simulink model "ModelanfisD"  (R2017a)
settings: Solver=VariableStepAuto  StartTime=0.0  StopTime=578  RelTol=1e-3
values from neighbouring files (symbols this model uses):
  dinneg12 = [-0.01 -0.01 -0.02 -0.01 -0.01 -0.01 0 0 0 0 0.01 -0.01 ... (2312 elements, 578x4)]    [anfisd.mat]    (also in anfisfin.mat; cinco.mat)
libraries: dspsrcs4 x77, fuzblock x22
settings Model: Creator=Dell  LastModifiedBy=Dell

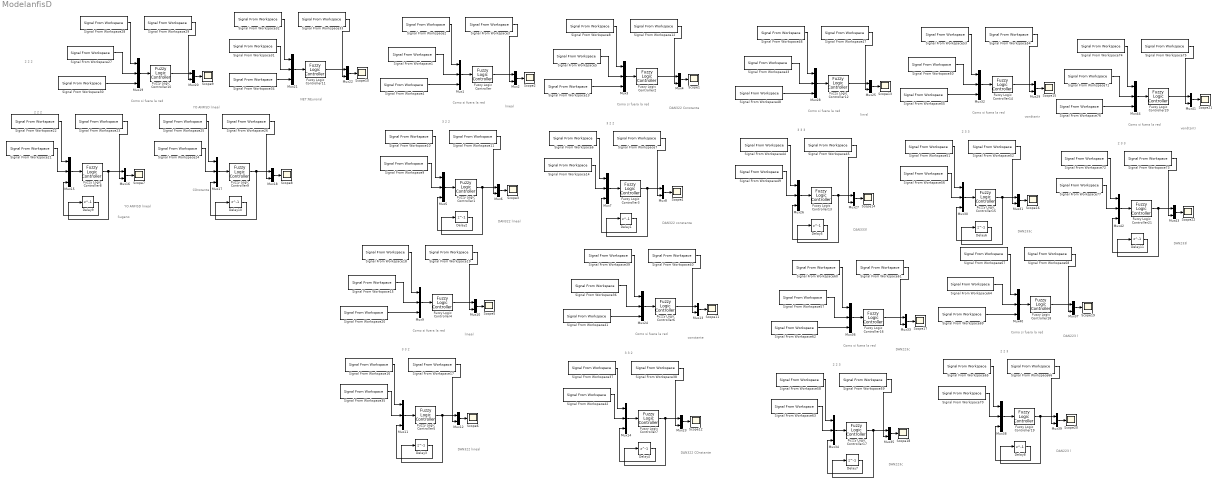
== system ModelanfisD ==
  note: lineal
  note: 3 2 2
  note: 2 2 2
  note: 2 2 2
  note: NET:NEuronal
  note: Como si fuera la red
  note: YO ANFISD lineal
  note: Sugeno
  note: COnstante
  note: YO ANFISD lineal
  note: Como si fuera la red
  note: DAN322 lineal
  note: DAN322 Constante
  note: 3 2 2
  note: Como si fuera la red
  note: DAN322 constante
  note: lineal
  note: 3 3 2
  note: Como si fuera la red
  note: DAN322 lineal
  note: constante
  note: 3 3 2
  note: Como si fuera la red
  note: DAN322 COnstante
  note: linrsl
  note: 3 3 3
  note: Como si fuera la red
  note: DAN333l
  note: vondtsntr
  note: 2 3 3
  note: Como si fuera la red
  note: DAN233c
  note: DAN223c
  note: 2 2 3
  note: Como si fuera la red
  note: DAN223c
  note: DAN223 l
  note: 2 2 3
  note: Como si fuera la red
  note: DAN223 l
  note: vondtsntr
  note: 2 3 3
  note: Como si fuera la red
  note: DAN233l
  Delay{1..11} (11 alike) : Delay  DelayLength=1
  Fuzzy Logic Controller : fuzblock/Fuzzy Logic  Controller  fis=DAN322ll
  Fuzzy Logic Controller1 : fuzblock/Fuzzy Logic  Controller  fis=DAN322ll
  Fuzzy Logic Controller10 : fuzblock/Fuzzy Logic  Controller  fis=ANFISD
  Fuzzy Logic Controller11 : fuzblock/Fuzzy Logic  Controller  fis=ANFISDC1
  Fuzzy Logic Controller12 : fuzblock/Fuzzy Logic  Controller  fis=DAN333l
  Fuzzy Logic Controller13 : fuzblock/Fuzzy Logic  Controller  fis=DAN333l
  Fuzzy Logic Controller14 : fuzblock/Fuzzy Logic  Controller  fis=DAN233
  Fuzzy Logic Controller15 : fuzblock/Fuzzy Logic  Controller  fis=DAN233
  Fuzzy Logic Controller16 : fuzblock/Fuzzy Logic  Controller  fis=DAN223
  Fuzzy Logic Controller17 : fuzblock/Fuzzy Logic  Controller  fis=DAN223
  Fuzzy Logic Controller18 : fuzblock/Fuzzy Logic  Controller  fis=DAN223l
  Fuzzy Logic Controller19 : fuzblock/Fuzzy Logic  Controller  fis=DAN223l
  Fuzzy Logic Controller2 : fuzblock/Fuzzy Logic  Controller  fis=DAN322c
  Fuzzy Logic Controller20 : fuzblock/Fuzzy Logic  Controller  fis=DAN233l
  Fuzzy Logic Controller21 : fuzblock/Fuzzy Logic  Controller  fis=DAN233l
  Fuzzy Logic Controller3 : fuzblock/Fuzzy Logic  Controller  fis=DAN322c
  Fuzzy Logic Controller4 : fuzblock/Fuzzy Logic  Controller  fis=DAN332
  Fuzzy Logic Controller5 : fuzblock/Fuzzy Logic  Controller  fis=DAN332
  Fuzzy Logic Controller6 : fuzblock/Fuzzy Logic  Controller  fis=DAN332c
  Fuzzy Logic Controller7 : fuzblock/Fuzzy Logic  Controller  fis=DAN332c
  Fuzzy Logic Controller8 : fuzblock/Fuzzy Logic  Controller  fis=ANFISD
  Fuzzy Logic Controller9 : fuzblock/Fuzzy Logic  Controller  fis=ANFISDC1
  Mux{1,3,5,7,9,11,14..15,17,19,21,24,26,28,30,32,34,36,38,40,42,44} (22 alike) : Mux  Inputs=3
  Mux{2,4,6,8,10,12..13,16,18,20,22..23,25,27,29,31,33,35,37,39,41,43} (22 alike) : Mux  Inputs=2
  Scope{1..22} (22 alike) : Scope
  Signal From Workspace{1,5,9,14..15,21,24,27,31,35..36,42..43,49..50,56..57,63..64,70..71,77} (22 alike) : dspsrcs4/Signal From Workspace  X=dinneg12(:,2)  Ts=1  nsamps=1  OutputAfterFinalValue=Setting to zero  ignoreOrWarnInputAndFrameLengths=off  OutputFrames=off
  Signal From Workspace{2,6,8,10,16,18,22,25,28,32,37,39,44,46,51,53,58,60,65,67,72,74} (22 alike) : dspsrcs4/Signal From Workspace  X=dinneg12(:,1)  Ts=1  nsamps=1  OutputAfterFinalValue=Setting to zero  ignoreOrWarnInputAndFrameLengths=off  OutputFrames=off
  Signal From Workspace{3,7,11..12,17,19,23,26,29,33,38,40,45,47,52,54,59,61,66,68,73,75} (22 alike) : dspsrcs4/Signal From Workspace  X=dinneg12(:,4)  Ts=1  nsamps=1  OutputAfterFinalValue=Setting to zero  ignoreOrWarnInputAndFrameLengths=off  OutputFrames=off
  Signal From Workspace{4,13,20,30,34,41,48,55,62,69,76} (11 alike) : dspsrcs4/Signal From Workspace  X=dinneg12(:,3)  Ts=1  nsamps=1  OutputAfterFinalValue=Setting to zero  ignoreOrWarnInputAndFrameLengths=off  OutputFrames=off
  wires:
  Signal From Workspace34/1 -> Mux21/3
  Signal From Workspace31/1 -> Mux21/2
  Signal From Workspace33/1 -> Mux22/2
  Signal From Workspace32/1 -> Mux21/1
  Mux22/1 -> Scope10/1
  Fuzzy Logic Controller11/1 -> Mux22/1
  Mux21/1 -> Fuzzy Logic Controller11/1
  Signal From Workspace30/1 -> Mux19/3
  Signal From Workspace27/1 -> Mux19/2
  Fuzzy Logic Controller10/1 -> Mux20/1
  Signal From Workspace28/1 -> Mux19/1
  Mux20/1 -> Scope9/1
  Signal From Workspace29/1 -> Mux20/2
  Mux19/1 -> Fuzzy Logic Controller10/1
  Mux17/1 -> Fuzzy Logic Controller9/1
  Fuzzy Logic Controller9/1 -> Mux18/1, Delay10/1
  Mux18/1 -> Scope8/1
  Signal From Workspace25/1 -> Mux17/1
  Signal From Workspace26/1 -> Mux18/2
  Delay10/1 -> Mux17/3
  Signal From Workspace24/1 -> Mux17/2
  Signal From Workspace21/1 -> Mux15/2
  Delay9/1 -> Mux15/3
  Signal From Workspace23/1 -> Mux16/2
  Signal From Workspace22/1 -> Mux15/1
  Mux16/1 -> Scope7/1
  Fuzzy Logic Controller8/1 -> Delay9/1, Mux16/1
  Mux15/1 -> Fuzzy Logic Controller8/1
  Mux1/1 -> Fuzzy Logic Controller/1
  Signal From Workspace3/1 -> Mux2/2
  Mux2/1 -> Scope2/1
  Signal From Workspace2/1 -> Mux1/1
  Fuzzy Logic Controller/1 -> Mux2/1
  Signal From Workspace1/1 -> Mux1/2
  Signal From Workspace4/1 -> Mux1/3
  Mux5/1 -> Fuzzy Logic Controller1/1
  Fuzzy Logic Controller1/1 -> Mux6/1, Delay2/1
  Mux6/1 -> Scope3/1
  Signal From Workspace10/1 -> Mux5/1
  Signal From Workspace11/1 -> Mux6/2
  Delay2/1 -> Mux5/3
  Signal From Workspace9/1 -> Mux5/2
  Signal From Workspace14/1 -> Mux7/2
  Delay1/1 -> Mux7/3
  Signal From Workspace7/1 -> Mux8/2
  Signal From Workspace6/1 -> Mux7/1
  Mux8/1 -> Scope4/1
  Fuzzy Logic Controller3/1 -> Delay1/1, Mux8/1
  Mux7/1 -> Fuzzy Logic Controller3/1
  Signal From Workspace13/1 -> Mux3/3
  Signal From Workspace5/1 -> Mux3/2
  Fuzzy Logic Controller2/1 -> Mux4/1
  Signal From Workspace8/1 -> Mux3/1
  Mux4/1 -> Scope1/1
  Signal From Workspace12/1 -> Mux4/2
  Mux3/1 -> Fuzzy Logic Controller2/1
  Signal From Workspace35/1 -> Mux11/2
  Delay3/1 -> Mux11/3
  Signal From Workspace17/1 -> Mux12/2
  Signal From Workspace16/1 -> Mux11/1
  Mux12/1 -> Scope6/1
  Fuzzy Logic Controller5/1 -> Delay3/1, Mux12/1
  Mux11/1 -> Fuzzy Logic Controller5/1
  Signal From Workspace20/1 -> Mux9/3
  Signal From Workspace15/1 -> Mux9/2
  Fuzzy Logic Controller4/1 -> Mux10/1
  Signal From Workspace18/1 -> Mux9/1
  Mux10/1 -> Scope5/1
  Signal From Workspace19/1 -> Mux10/2
  Mux9/1 -> Fuzzy Logic Controller4/1
  Mux24/1 -> Fuzzy Logic Controller6/1
  Signal From Workspace40/1 -> Mux13/2
  Mux13/1 -> Scope11/1
  Signal From Workspace39/1 -> Mux24/1
  Fuzzy Logic Controller6/1 -> Mux13/1
  Signal From Workspace36/1 -> Mux24/2
  Signal From Workspace41/1 -> Mux24/3
  Mux14/1 -> Fuzzy Logic Controller7/1
  Fuzzy Logic Controller7/1 -> Mux23/1, Delay4/1
  Mux23/1 -> Scope12/1
  Signal From Workspace37/1 -> Mux14/1
  Signal From Workspace38/1 -> Mux23/2
  Delay4/1 -> Mux14/3
  Signal From Workspace42/1 -> Mux14/2
  Signal From Workspace49/1 -> Mux26/2
  Delay5/1 -> Mux26/3
  Signal From Workspace45/1 -> Mux27/2
  Signal From Workspace44/1 -> Mux26/1
  Mux27/1 -> Scope14/1
  Fuzzy Logic Controller13/1 -> Delay5/1, Mux27/1
  Mux26/1 -> Fuzzy Logic Controller13/1
  Signal From Workspace48/1 -> Mux28/3
  Signal From Workspace43/1 -> Mux28/2
  Fuzzy Logic Controller12/1 -> Mux25/1
  Signal From Workspace46/1 -> Mux28/1
  Mux25/1 -> Scope13/1
  Signal From Workspace47/1 -> Mux25/2
  Mux28/1 -> Fuzzy Logic Controller12/1
  Mux32/1 -> Fuzzy Logic Controller14/1
  Signal From Workspace54/1 -> Mux29/2
  Mux29/1 -> Scope15/1
  Signal From Workspace53/1 -> Mux32/1
  Fuzzy Logic Controller14/1 -> Mux29/1
  Signal From Workspace50/1 -> Mux32/2
  Signal From Workspace55/1 -> Mux32/3
  Mux30/1 -> Fuzzy Logic Controller15/1
  Fuzzy Logic Controller15/1 -> Mux31/1, Delay6/1
  Mux31/1 -> Scope16/1
  Signal From Workspace51/1 -> Mux30/1
  Signal From Workspace52/1 -> Mux31/2
  Delay6/1 -> Mux30/3
  Signal From Workspace56/1 -> Mux30/2
  Signal From Workspace63/1 -> Mux34/2
  Delay7/1 -> Mux34/3
  Signal From Workspace59/1 -> Mux35/2
  Signal From Workspace58/1 -> Mux34/1
  Mux35/1 -> Scope18/1
  Fuzzy Logic Controller17/1 -> Delay7/1, Mux35/1
  Mux34/1 -> Fuzzy Logic Controller17/1
  Signal From Workspace62/1 -> Mux36/3
  Signal From Workspace57/1 -> Mux36/2
  Fuzzy Logic Controller16/1 -> Mux33/1
  Signal From Workspace60/1 -> Mux36/1
  Mux33/1 -> Scope17/1
  Signal From Workspace61/1 -> Mux33/2
  Mux36/1 -> Fuzzy Logic Controller16/1
  Mux40/1 -> Fuzzy Logic Controller18/1
  Signal From Workspace68/1 -> Mux37/2
  Mux37/1 -> Scope19/1
  Signal From Workspace67/1 -> Mux40/1
  Fuzzy Logic Controller18/1 -> Mux37/1
  Signal From Workspace64/1 -> Mux40/2
  Signal From Workspace69/1 -> Mux40/3
  Mux38/1 -> Fuzzy Logic Controller19/1
  Fuzzy Logic Controller19/1 -> Mux39/1, Delay8/1
  Mux39/1 -> Scope20/1
  Signal From Workspace65/1 -> Mux38/1
  Signal From Workspace66/1 -> Mux39/2
  Delay8/1 -> Mux38/3
  Signal From Workspace70/1 -> Mux38/2
  Signal From Workspace77/1 -> Mux42/2
  Delay11/1 -> Mux42/3
  Signal From Workspace73/1 -> Mux43/2
  Signal From Workspace72/1 -> Mux42/1
  Mux43/1 -> Scope22/1
  Fuzzy Logic Controller21/1 -> Delay11/1, Mux43/1
  Mux42/1 -> Fuzzy Logic Controller21/1
  Signal From Workspace76/1 -> Mux44/3
  Signal From Workspace71/1 -> Mux44/2
  Fuzzy Logic Controller20/1 -> Mux41/1
  Signal From Workspace74/1 -> Mux44/1
  Mux41/1 -> Scope21/1
  Signal From Workspace75/1 -> Mux41/2
  Mux44/1 -> Fuzzy Logic Controller20/1
